simulink model "recursive_running_sum_3"  (R2014b)
settings: Solver=ode45  StartTime=0.0  StopTime=inf  RelTol=1e-3
undefined symbols (not defined in the file or in its folder): filtk, filtk3
libraries: simulink x1
settings Model: Creator=Ben  LastModifiedBy=Ben

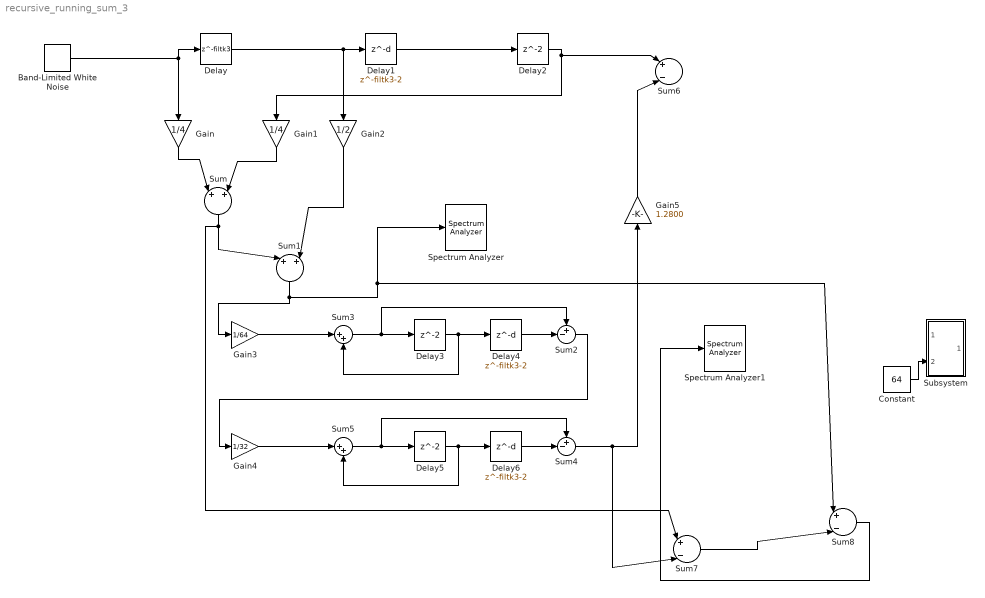
== system recursive_running_sum_3 ==
  Band-Limited White Noise : simulink/Sources/Band-Limited White Noise  Cov=[0.01]  Ts=1/200  seed=[23341]
  Constant : Constant  Value=64
  Delay : Delay  DelayLength=filtk3  InitialCondition=0
  Delay1 : Delay  DelayLength=filtk3-2  InitialCondition=0
  Delay2 : Delay  InitialCondition=0
  Delay3 : Delay  InitialCondition=0
  Delay4 : Delay  DelayLength=filtk3-2  InitialCondition=0
  Delay5 : Delay  InitialCondition=0
  Delay6 : Delay  DelayLength=filtk3-2  InitialCondition=0
  Gain : Gain  Gain=1/4
  Gain1 : Gain  Gain=1/4
  Gain2 : Gain  Gain=1/2
  Gain3 : Gain  Gain=1/64
  Gain4 : Gain  Gain=1/32
  Gain5 : Gain  Gain=1.2800
  Spectrum Analyzer : SpectrumAnalyzer
  Spectrum Analyzer1 : SpectrumAnalyzer
  Subsystem : Subsystem
  Sum : Sum  Inputs=|+|+|
  Sum1 : Sum  Inputs=|+|+|
  Sum2 : Sum  Inputs=+-|
  Sum3 : Sum  Inputs=|++
  Sum4 : Sum  Inputs=+-|
  Sum5 : Sum  Inputs=|++
  Sum6 : Sum  Inputs=|+|-|
  Sum7 : Sum  Inputs=|+|-|
  Sum8 : Sum  Inputs=|+|-|
  wires:
  Delay/1 -> Gain2/1, Delay1/1
  Delay1/1 -> Delay2/1
  Gain1/1 -> Sum/2
  Gain/1 -> Sum/1
  Delay2/1 -> Gain1/1, Sum6/1
  Sum/1 -> Sum7/1, Sum1/1
  Gain2/1 -> Sum1/2
  Gain4/1 -> Sum5/1
  Sum5/1 -> Sum4/1, Delay5/1
  Delay5/1 -> Delay6/1, Sum5/2
  Delay6/1 -> Sum4/2
  Sum4/1 -> Sum7/2, Gain5/1
  Band-Limited White Noise/1 -> Gain/1, Delay/1
  Constant/1 -> Subsystem/2(In2)
  Sum1/1 -> Sum8/1, Spectrum Analyzer/1, Gain3/1
  Gain3/1 -> Sum3/1
  Sum3/1 -> Sum2/1, Delay3/1
  Delay3/1 -> Delay4/1, Sum3/2
  Delay4/1 -> Sum2/2
  Sum2/1 -> Gain4/1
  Gain5/1 -> Sum6/2
  Sum7/1 -> Sum8/2
  Sum8/1 -> Spectrum Analyzer1/1

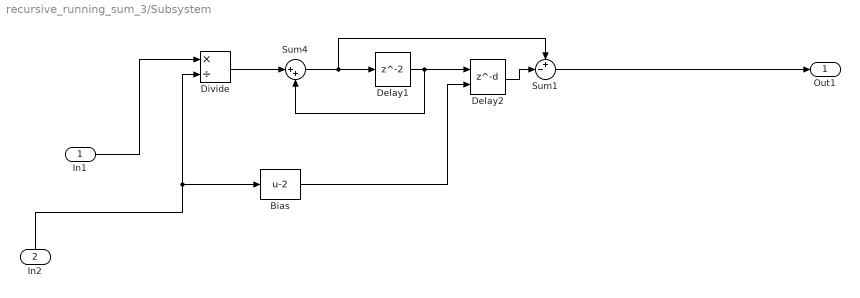
== system recursive_running_sum_3/Subsystem ==
  In1 : Inport
  In2 : Inport  Port=2
  Bias : Bias  Bias=-2
  Delay1 : Delay  InitialCondition=0
  Delay2 : Delay  DelayLengthSource=Input port  DelayLength=filtk-1  InitialCondition=0
      settings: InputPortMap=u0,p1
  Divide : Product  Inputs=*/
  Sum1 : Sum  Inputs=+-|
  Sum4 : Sum  Inputs=|++
  Out1 : Outport
  wires:
  Sum4/1 -> Sum1/1, Delay1/1
  Delay1/1 -> Delay2/1, Sum4/2
  Delay2/1 -> Sum1/2
  Sum1/1 -> Out1/1
  In1/1 -> Divide/1
  Divide/1 -> Sum4/1
  Bias/1 -> Delay2/2
  In2/1 -> Divide/2, Bias/1
